simulink model "AUV_Model"  (R2020a)
settings: Solver=VariableStepAuto  StartTime=0.0  StopTime=300  FixedStep=0.5  RelTol=1e-3
InitFcn:
  | mdlWks = get_param(gcs,'ModelWorkspace');
  | a = getVariable(mdlWks,'a');
  | b = getVariable(mdlWks,'b');
  | c = getVariable(mdlWks,'c');
StopFcn:
  | figure(2)
  | plot3(Position_Data(1,1),Position_Data(1,2),Position_Data(1,3),'r*')
  | hold on
  | plot3(Position_Data(:,1),Position_Data(:,2),Position_Data(:,3));
  | plot3(Position_Data(end,1),Position_Data(end,2),Position_Data(end,3),'g*');
  | grid on
  | legend('Start Point','Trajectory','End Point')
model workspace (MAT data in the model file):
  a = 0
  b = 1
  c = 1
undefined symbols (not defined in the file or in its folder): sigbuilder_block
libraries: dspfdesign x6, mpclib x1, aerolibnav x1
(part 2 of 2)

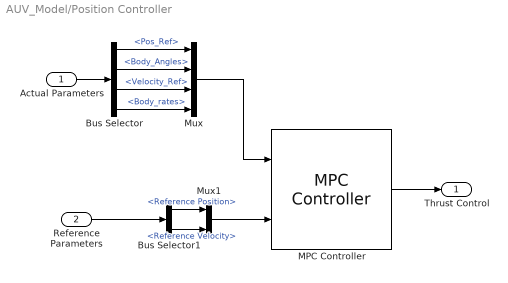
== system AUV_Model/Position Controller ==
  Actual Parameters : Inport
  Reference Parameters : Inport  Port=2
  Bus Selector : BusSelector  OutputSignals=Pos_Ref,Body_Angles,Velocity_Ref,Body_rates
  Bus Selector1 : BusSelector  OutputSignals=Reference Position,Reference Velocity
  MPC Controller : mpclib/MPC Controller  SCDEnableBlockLinearizationSpecification=on  mpcobj=mpc1  is_multiple=0  enable_value=0  return_u0=off  updateMPCinCallerWorkspace=on  md_inport=off  mv_inport=off  uref_inport=off  return_cost=off  return_mvseq=off  return_qpstatus=off  return_xseq=off  return_state=off  return_ovseq=off  state_inport=off  umin_inport=off  umax_inport=off  ymin_inport=off  ymax_inport=off  cc_inport=off  ywt_inport=off  uwt_inport=off  duwt_inport=off  rhoeps_inport=off  pm_inport=off  MaximumP=10  HorizonChoice=FixedHorizon  n_ts=0.1  n_p=10  n_mv=8  n_md=0  n_ud=0  n_mo=12  n_uo=0  BlockDataType=double  SampleTimeInherited=off  switch_inport=off
  Mux : Mux
  Mux1 : Mux  Inputs=2
  Thrust Control : Outport  VectorParamsAs1DForOutWhenUnconnected=off
  wires:
  Actual Parameters/1 -> Bus Selector/1
  MPC Controller/1 -> Thrust Control/1
  Mux/1 -> MPC Controller/1
  Bus Selector/1 -> Mux/1  "<Pos_Ref>"
  Bus Selector/2 -> Mux/2  "<Body_Angles>"
  Bus Selector1/1 -> Mux1/1  "<Reference Position>"
  Reference Parameters/1 -> Bus Selector1/1
  Mux1/1 -> MPC Controller/2
  Bus Selector1/2 -> Mux1/2  "<Reference Velocity>"
  Bus Selector/3 -> Mux/3  "<Velocity_Ref>"
  Bus Selector/4 -> Mux/4  "<Body_rates>"

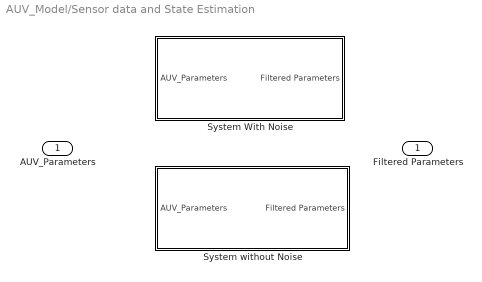
== system AUV_Model/Sensor data and State Estimation ==
  AUV_Parameters : Inport
  System With Noise : Subsystem  VariantControl=b==0
  System without Noise : Subsystem  VariantControl=b==1
  Filtered Parameters : Outport  VectorParamsAs1DForOutWhenUnconnected=off

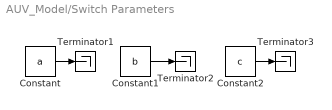
== system AUV_Model/Switch Parameters ==
  Constant : Constant  Value=a
  Constant1 : Constant  Value=b
  Constant2 : Constant  Value=c
  Terminator1 : Terminator
  Terminator2 : Terminator
  Terminator3 : Terminator
  wires:
  Constant/1 -> Terminator1/1
  Constant1/1 -> Terminator2/1
  Constant2/1 -> Terminator3/1

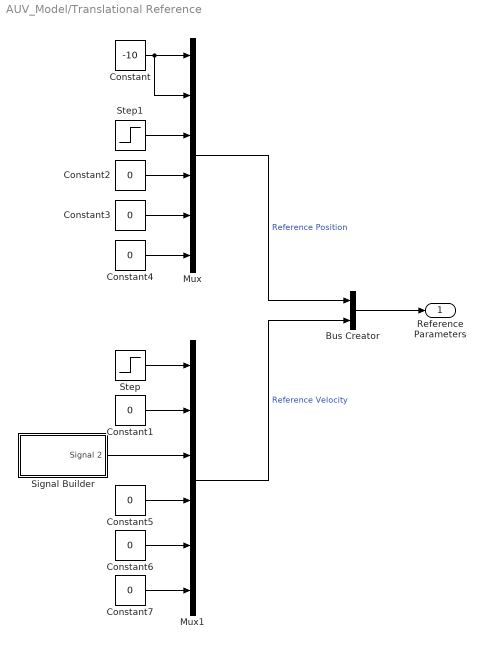
== system AUV_Model/Translational Reference ==
  Bus Creator : BusCreator  Inputs=2
  Constant : Constant  Value=-10
  Constant{1..7} (7 alike) : Constant  Value=0
  Mux : Mux  Inputs=6
  Mux1 : Mux  Inputs=6
  Signal Builder : Subsystem  Tag=STV Subsys  LoadFcn=sigbuilder_block('load');  StartFcn=sigbuilder_block('start');  StopFcn=sigbuilder_block('stop');  ClipboardFcn=sigbuilder_block('clipboard');  mask(Sigbuilder block){tuvar=[0:10]}
      mask help: Simulink:masks:SigbuilderBlock_MD
      mask init:
      | if ~strcmp(get_param(bdroot(gcbh),'SimulationStatus'),'stopped') tuvar = sigbuilder_block('maskInit'); end
      settings: CopyFcn=sigbuilder_block('copy');  DeleteFcn=sigbuilder_block('delete');  ModelCloseFcn=sigbuilder_block('modelClose');  PreSaveFcn=sigbuilder_block('preSave');  PauseFcn=sigbuilder_block('pause');  ContinueFcn=sigbuilder_block('continue');  NameChangeFcn=sigbuilder_block('namechange');  OpenFcn=sigbuilder_block('open',[357.5 219 1204.5 357 ]);  CloseFcn=sigbuilder_block('close');
      mask Display: plot(0, 0, 100, 100,[2, 2, 32, 32, 2], [68, 8, 8, 68, 68],[32, 2], [38, 38], [32, 19, 2],[53, 60, 44], [32, 17, 17, 2],[16, 16, 31, 31]);txt = getActiveGroup(gcbh);text(2, 100, txt,'verticalAlignment', 'top');
  Step : Step  Time=30  Before=0.2  After=0  SampleTime=0
  Step1 : Step  Time=150  After=5  SampleTime=0
  Reference Parameters : Outport  VectorParamsAs1DForOutWhenUnconnected=off
  wires:
  Mux/1 -> Bus Creator/1  "Reference Position"
  Constant/1 -> Mux/2, Mux/1
  Step1/1 -> Mux/3
  Mux1/1 -> Bus Creator/2  "Reference Velocity"
  Bus Creator/1 -> Reference Parameters/1
  Signal Builder/1(Signal 2) -> Mux1/3
  Constant1/1 -> Mux1/2
  Step/1 -> Mux1/1
  Constant2/1 -> Mux/4
  Constant3/1 -> Mux/5
  Constant4/1 -> Mux/6
  Constant6/1 -> Mux1/5
  Constant7/1 -> Mux1/6
  Constant5/1 -> Mux1/4

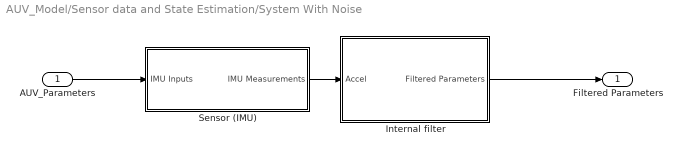
== system AUV_Model/Sensor data and State Estimation/System With Noise ==
  AUV_Parameters : Inport
  " Sensor (IMU)" : Subsystem
  Internal filter : Subsystem
  Filtered Parameters : Outport  VectorParamsAs1DForOutWhenUnconnected=off
  wires:
  AUV_Parameters/1 -> " Sensor (IMU)"/1(IMU Inputs)
  Internal filter/1(Filtered Parameters) -> Filtered Parameters/1
  " Sensor (IMU)"/1(IMU Measurements) -> Internal filter/1(Accel)

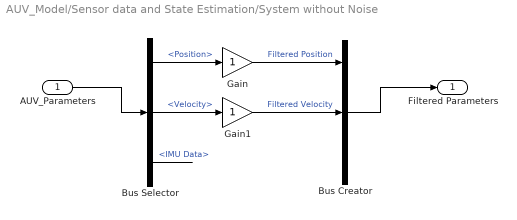
== system AUV_Model/Sensor data and State Estimation/System without Noise ==
  AUV_Parameters : Inport
  Bus Creator : BusCreator  Inputs=3
  Bus Selector : BusSelector  OutputSignals=Position,Velocity,IMU Data
  Gain : Gain
  Gain1 : Gain
  Filtered Parameters : Outport  VectorParamsAs1DForOutWhenUnconnected=off
  wires:
  Bus Creator/1 -> Filtered Parameters/1
  Bus Selector/2 -> Gain1/1  "<Velocity>"
  Bus Selector/1 -> Gain/1  "<Position>"
  Gain1/1 -> Bus Creator/2  "Filtered Velocity"
  Gain/1 -> Bus Creator/1  "Filtered Position"
  AUV_Parameters/1 -> Bus Selector/1
  Bus Selector/3 -> ?  "<IMU Data>"

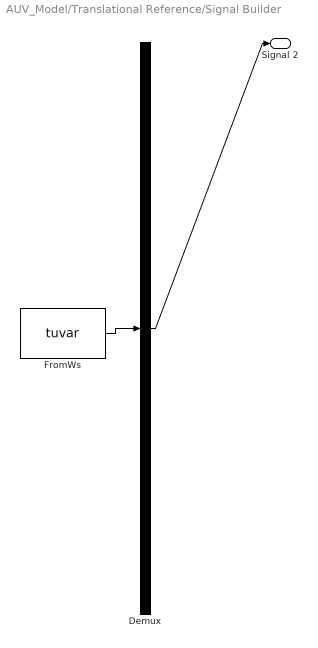
== system AUV_Model/Translational Reference/Signal Builder ==
  Demux : Demux  Tag=STV Demux  Outputs=1
      settings: DisplayOption=none
  FromWs : FromWorkspace  Tag=STV FromWs  VariableName=tuvar
      SigBuilderData=|
      | common.afterFinalStr = 'Extrapolate'
      | common.sampleTime = 0
      | dataSet.timeRange = [0 300]
      | dataSet.name = 'Group 1'
      | sbobj.Groups.Name = 'Group 1'
      | sbobj.Groups.Signals.Name = 'Signal 2'
      | sbobj.Groups.Signals.XData = [0 150 150 180 180 300]
      | sbobj.Groups.Signals.YData = [0 0 0.2 0.2 0 0]
      | sbobj.Groups.TimeRange = [0 300]
  Signal 2 : Outport  Tag=STV Outport  VectorParamsAs1DForOutWhenUnconnected=off
  wires:
  FromWs/1 -> Demux/1
  Demux/1 -> Signal 2/1

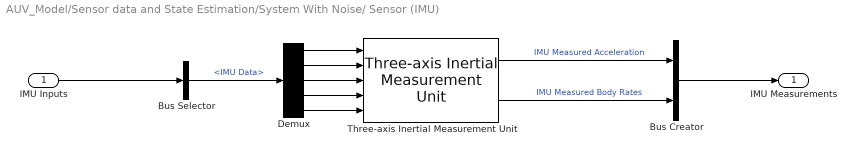
== system AUV_Model/Sensor data and State Estimation/System With Noise/ Sensor (IMU) ==
  IMU Inputs : Inport
  Bus Creator : BusCreator  Inputs=2
  Bus Selector : BusSelector  OutputSignals=IMU Data
  Demux : Demux  Outputs=5
  Three-axis Inertial Measurement Unit : aerolibnav/Three-axis Inertial Measurement Unit  units=Metric (MKS)  imu=[0 0 0]  i_Ts=0  dtype_a=on  w_a=190  z_a=0.707  a_sf_cc=[1 0 0; 0 1 0; 0 0 1]  a_bias=[0 0 0]  a_sat="[-inf  -inf  -inf  inf inf inf]"  dtype_g=on  w_g=190  z_g=0.707  g_sf_cc=[1 0 0; 0 1 0; 0 0 1]  g_bias=[0 0 0]  g_sens=[0 0 0]  g_sat="[-inf  -inf  -inf  inf inf inf]"  i_rand=on  i_seeds=[23093 23094 23095 23096 23097 23098]  i_pow=[0.00001 0.00001 0.00001 0.00001 0.00001 0.00001]
  IMU Measurements : Outport  VectorParamsAs1DForOutWhenUnconnected=off
  wires:
  Three-axis Inertial Measurement Unit/1 -> Bus Creator/1  "IMU Measured Acceleration"
  Demux/2 -> Three-axis Inertial Measurement Unit/2
  Demux/4 -> Three-axis Inertial Measurement Unit/4
  Demux/5 -> Three-axis Inertial Measurement Unit/5
  Demux/3 -> Three-axis Inertial Measurement Unit/3
  Demux/1 -> Three-axis Inertial Measurement Unit/1
  Three-axis Inertial Measurement Unit/2 -> Bus Creator/2  "IMU Measured Body Rates"
  IMU Inputs/1 -> Bus Selector/1
  Bus Selector/1 -> Demux/1  "<IMU Data>"
  Bus Creator/1 -> IMU Measurements/1

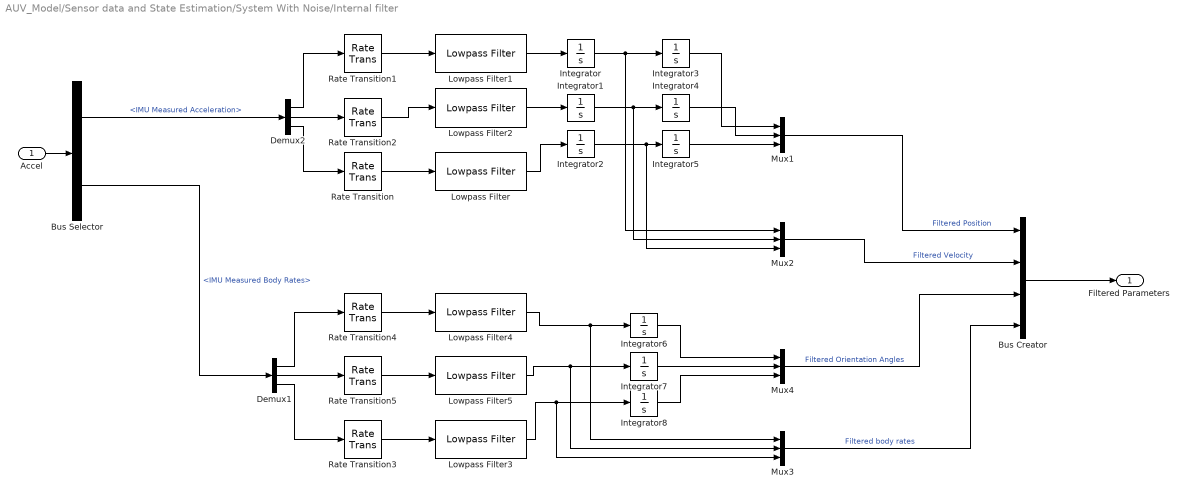
== system AUV_Model/Sensor data and State Estimation/System With Noise/Internal filter ==
  Accel : Inport
  Bus Creator : BusCreator  Inputs=4
  Bus Selector : BusSelector  OutputSignals=IMU Measured Acceleration,IMU Measured Body Rates
  Demux1 : Demux  Outputs=3
  Demux2 : Demux  Outputs=3
  Integrator{,1..8} (9 alike) : Integrator
  Lowpass Filter{,1..5} (6 alike) : dspfdesign/Lowpass Filter  FilterType=FIR  DesignForMinimumOrder=on  FilterOrder=50  PassbandFrequency=1/100  StopbandFrequency=45  PassbandRipple=0.1  StopbandAttenuation=80  InheritSampleRate=off  SampleRate=100  SimulateUsing=Interpreted execution  roundingMode=Floor  coeffsDataTypeStr=fixdt(1,16)
  Mux{1..4} (4 alike) : Mux  Inputs=3
  Rate Transition{,1..5} (6 alike) : RateTransition  OutPortSampleTime=0.01
  Filtered Parameters : Outport  VectorParamsAs1DForOutWhenUnconnected=off
  wires:
  Rate Transition5/1 -> Lowpass Filter5/1
  Rate Transition4/1 -> Lowpass Filter4/1
  Demux1/1 -> Rate Transition4/1
  Lowpass Filter3/1 -> Mux3/3, Integrator8/1
  Demux1/2 -> Rate Transition5/1
  Lowpass Filter5/1 -> Mux3/2, Integrator7/1
  Lowpass Filter4/1 -> Mux3/1, Integrator6/1
  Integrator6/1 -> Mux4/1
  Rate Transition3/1 -> Lowpass Filter3/1
  Integrator8/1 -> Mux4/3
  Demux1/3 -> Rate Transition3/1
  Integrator7/1 -> Mux4/2
  Accel/1 -> Bus Selector/1
  Bus Selector/1 -> Demux2/1  "<IMU Measured Acceleration>"
  Bus Selector/2 -> Demux1/1  "<IMU Measured Body Rates>"
  Mux4/1 -> Bus Creator/3  "Filtered Orientation Angles"
  Mux3/1 -> Bus Creator/4  "Filtered body rates"
  Bus Creator/1 -> Filtered Parameters/1
  Integrator2/1 -> Integrator5/1, Mux2/3
  Integrator/1 -> Mux2/1, Integrator3/1
  Mux2/1 -> Bus Creator/2  "Filtered Velocity"
  Mux1/1 -> Bus Creator/1  "Filtered Position"
  Lowpass Filter/1 -> Integrator2/1
  Demux2/2 -> Rate Transition2/1
  Rate Transition1/1 -> Lowpass Filter1/1
  Integrator4/1 -> Mux1/2
  Demux2/3 -> Rate Transition/1
  Lowpass Filter2/1 -> Integrator1/1
  Lowpass Filter1/1 -> Integrator/1
  Demux2/1 -> Rate Transition1/1
  Integrator5/1 -> Mux1/3
  Integrator1/1 -> Integrator4/1, Mux2/2
  Rate Transition/1 -> Lowpass Filter/1
  Integrator3/1 -> Mux1/1
  Rate Transition2/1 -> Lowpass Filter2/1
